simulink model "FMS_Simulation"  (R2024b)
settings: Solver=FixedStepDiscrete  StartTime=0.0  StopTime=100.0  FixedStep=0.1  RelTol=1e-3
settings Model: Creator=emilienboissy  LastModifiedBy=emilienboissy

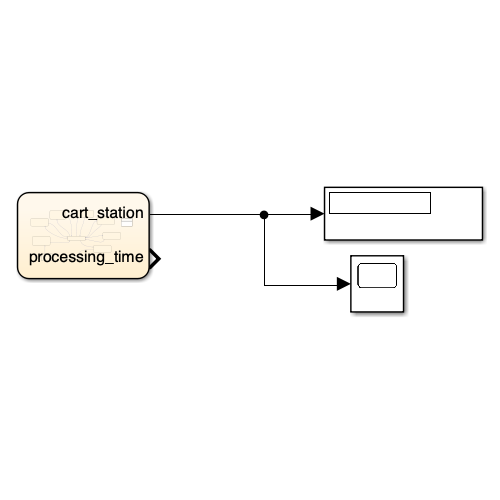
[thumbnail: Simulink's stored preview of the top-level diagram]
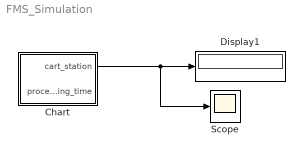
== system FMS_Simulation ==
  Chart : Stateflow chart  TreatAsAtomicUnit=on
  Display1 : Display
  Scope : Scope
  wires:
  Chart/1(cart_station) -> Scope/1, Display1/1

== stateflow chart FMS_Simulation/Chart ==
  state Station3
    entry: cart_station = 3;
    elapsed = 0;
    send_mqtt(3, 'CART_IN');
    during: elapsed = elapsed + 0.1;
    exit: send_mqtt(3, 'DONE');
  state Station4
    entry: cart_station = 4;
    elapsed = 0;
    send_mqtt(4, 'CART_IN');
    during: elapsed = elapsed + 0.1;
    exit: send_mqtt(4, 'DONE');
  state Station5
    entry: cart_station = 5;
    elapsed = 0;
    send_mqtt(5, 'CART_IN');
    during: elapsed = elapsed + 0.1;
    exit: send_mqtt(5, 'DONE');
  state Station2
    entry: cart_station = 2;
    elapsed = 0;
    send_mqtt(2, 'CART_IN');
    during: elapsed = elapsed + 0.1;
    exit: send_mqtt(2, 'DONE');
  state Station6
    entry: cart_station = 6;
    elapsed = 0;
    send_mqtt(6, 'CART_IN');
    during: elapsed = elapsed + 0.1;
    exit: send_mqtt(6, 'DONE');
  state MOVING
    entry: elapsed = 0;
    during: elapsed = elapsed + 0.1;
  state Station1
    entry: cart_station = 1; elapsed = 0;
    send_mqtt(1, 'CART_IN');
    during: elapsed = elapsed + 0.1;
    exit: send_mqtt(1, 'DONE');
  state Station7
    entry: cart_station = 7;
    elapsed = 0;
    send_mqtt(7, 'CART_IN');
    during: elapsed = elapsed + 0.1;
    exit: send_mqtt(7, 'DONE');
  state IDLE
    entry:
    dt =0.1; cart_station = 0;
    processing_time = 0;
    elapsed = 0;
    during: elapsed = elapsed + 0.1;
  state FINISHED
    entry: cart_station = 8;
    send_mqtt(0, 'FINISHED');
  Station3 -> MOVING : [elapsed >= 5]/{elapsed = 0;}
  MOVING -> Station3 [order 2] : [elapsed >= 2 && cart_station == 2]
  MOVING -> Station4 [order 4] : [elapsed >= 2 && cart_station == 3]
  Station4 -> MOVING : [elapsed >= 5]/{elapsed = 0;}
  MOVING -> Station5 [order 5] : [elapsed >= 2 && cart_station == 4]
  Station2 -> MOVING : [elapsed >= 5]/{elapsed = 0;}
  Station5 -> MOVING : [elapsed >= 5]/{elapsed = 0;}
  MOVING -> Station2 [order 1] : [elapsed >= 2 && cart_station == 1]
  MOVING -> Station6 [order 6] : [elapsed >= 2 && cart_station == 5]
  Station6 -> MOVING : [elapsed >= 5]/{elapsed = 0;}
  Station1 -> MOVING : [elapsed >= 5]/{elapsed = 0;}
  MOVING -> Station7 [order 3] : [elapsed >= 2 && cart_station == 6]
  IDLE -> Station1 : [elapsed >= 1]/{elapsed = 0;}
  Station7 -> FINISHED : [elapsed >= 5]/{elapsed = 0;}
  (default) -> IDLE
  data: station function_input; signal function_input; dt local =0.1; cart_station output; processing_time output; elapsed local =0
  function send_mqtt(station, signal):
    | function send_mqtt(station, signal)
    | cmd = sprintf('/opt/homebrew/bin/python3.11 /Users/emilienboissy/Documents/DT-FMS/matlab_mqtt_send.py %d %s', station, signal);
    | system(cmd);
    | 
    | if strcmp(signal, 'CART_IN')
    |     wait_cmd = '/opt/homebrew/bin/python3.11 /Users/emilienboissy/Documents/DT-FMS/matlab_mqtt_wait.py';
    |     system(wait_cmd);
    | end
